simulink model "QuaternionFeedbackControl"  (R2024a)
settings: Solver=ode4  StartTime=0.0  StopTime=1000  FixedStep=0.5  RelTol=1e-3
libraries: aerolibutil x3, matrix_library x1
settings Model: Creator=dani  LastModifiedBy=dani

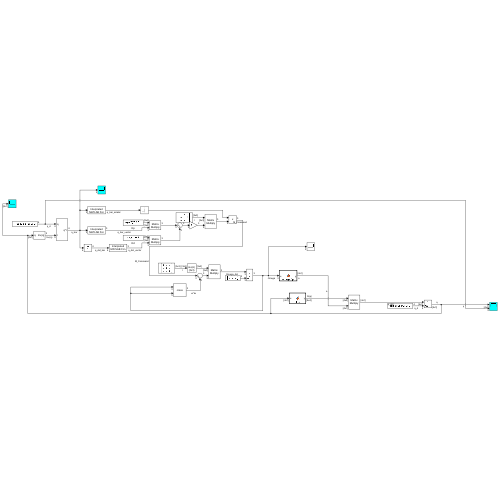
[thumbnail: Simulink's stored preview of the top-level diagram]
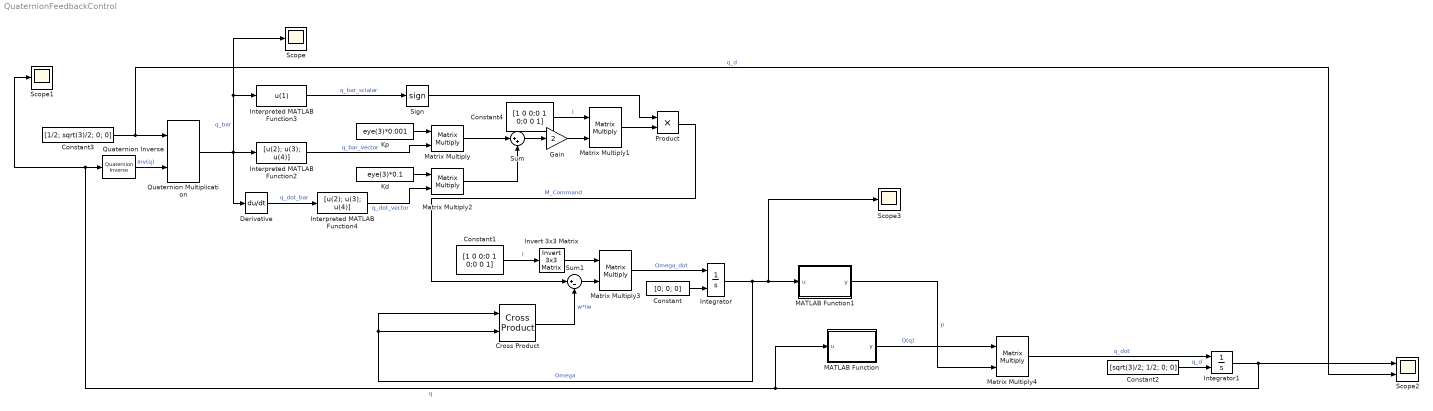
== system QuaternionFeedbackControl ==
  Constant : Constant  Value=[0; 0; 0]
  Constant1 : Constant  Value=[1 0 0;0 1 0;0 0 1]
  Constant2 : Constant  Value=[sqrt(3)/2; 1/2; 0; 0]
  Constant3 : Constant  Value=[1/2; sqrt(3)/2; 0; 0]
  Constant4 : Constant  Value=[1 0 0;0 1 0;0 0 1]
  Cross Product : matrix_library/Cross Product
  Derivative : Derivative
  Gain : Gain  Gain=2
  Integrator : Integrator  InitialConditionSource=external
  Integrator1 : Integrator  InitialConditionSource=external
  Interpreted MATLAB Function2 : MATLABFcn  MATLABFcn=[u(2); u(3); u(4)]
  Interpreted MATLAB Function3 : MATLABFcn  MATLABFcn=u(1)
  Interpreted MATLAB Function4 : MATLABFcn  MATLABFcn=[u(2); u(3); u(4)]
  Invert 3x3 Matrix : aerolibutil/Invert  3x3 Matrix
  Kd : Constant  Value=eye(3)*0.1
  Kp : Constant  Value=eye(3)*0.001
  MATLAB Function : MATLAB Function  TreatAsAtomicUnit=on
  MATLAB Function1 : MATLAB Function  TreatAsAtomicUnit=on
  Matrix Multiply{,1..4} (5 alike) : Product  Multiplication=Matrix(*)
  Product : Product
  Quaternion Inverse : aerolibutil/Quaternion Inverse
  Quaternion Multiplication : aerolibutil/Quaternion Multiplication
  Scope : Scope
  Scope1 : Scope
  Scope2 : Scope  NumInputPorts=2
  Scope3 : Scope
  Sign : Signum
  Sum : Sum  Inputs=|++
  Sum1 : Sum  Inputs=|+-
  wires:
  Constant1/1 -> Invert 3x3 Matrix/1  "I"
  Matrix Multiply3/1 -> Integrator/1  "Omega_dot"
  Integrator/1 -> Cross Product/2, Cross Product/1, Scope3/1, MATLAB Function1/1(u)  "Omega"
  Constant/1 -> Integrator/2
  Matrix Multiply4/1 -> Integrator1/1  "q_dot"
  Integrator1/1 -> Scope2/1, MATLAB Function/1(u), Quaternion Inverse/1, Scope1/1  "q"
  Constant2/1 -> Integrator1/2  "q_d"
  MATLAB Function/1(y) -> Matrix Multiply4/1  "Q(q)"
  MATLAB Function1/1(y) -> Matrix Multiply4/2  "p"
  Quaternion Multiplication/1 -> Scope/1, Interpreted MATLAB Function3/1, Derivative/1, Interpreted MATLAB Function2/1  "q_bar"
  Constant3/1 -> Scope2/2, Quaternion Multiplication/1  "q_d"
  Quaternion Inverse/1 -> Quaternion Multiplication/2  "Inv(q)"
  Interpreted MATLAB Function2/1 -> Matrix Multiply/2  "q_bar_vector"
  Interpreted MATLAB Function3/1 -> Sign/1  "q_bar_sclalar"
  Constant4/1 -> Matrix Multiply1/1  "I"
  Kp/1 -> Matrix Multiply/1
  Kd/1 -> Matrix Multiply2/1
  Derivative/1 -> Interpreted MATLAB Function4/1  "q_dot_bar"
  Matrix Multiply2/1 -> Sum/2
  Matrix Multiply/1 -> Sum/1
  Sum/1 -> Gain/1
  Matrix Multiply1/1 -> Product/2
  Sign/1 -> Product/1
  Product/1 -> Sum1/1  "M_Command"
  Invert 3x3 Matrix/1 -> Matrix Multiply3/1
  Interpreted MATLAB Function4/1 -> Matrix Multiply2/2  "q_dot_vector"
  Cross Product/1 -> Sum1/2  "w*Iw"
  Sum1/1 -> Matrix Multiply3/2
  Gain/1 -> Matrix Multiply1/2

== matlab function QuaternionFeedbackControl/MATLAB Function ==
  data: u input; y output
function y = qtoQ(u)

y = [u(1) -u(2) -u(3) -u(4); u(2) u(1) -u(4) u(3); u(3) u(4) u(1) -u(2); u(4) -u(3) u(2) u(1)];
end

== matlab function QuaternionFeedbackControl/MATLAB Function1 ==
  data: u input; y output
function y = omega2p(u)

y = [0; u(1); u(2); u(3)];
end
